simulink model "Lgsvl_ADRC_PP"  (R2023a)
settings: Solver=VariableStepAuto  StartTime=0.0  StopTime=inf  RelTol=1e-3
values from neighbouring files (symbols this model uses):
  Caf = 140000    [ADRC_PP.m]    (also in ADRC_Pure_Pursuit.m)
  Izz = 1000    [ADRC_PP.m]    (also in ADRC_Pure_Pursuit.m)
  lf = 1.63886    [ADRC_PP.m]    (also in ADRC_Pure_Pursuit.m)
  observer_discrete = c2d(observer, T)    [ADRC_PP.m]    (also in ADRC_Pure_Pursuit.m)
libraries: ros2lib x8, simulink_extras x2
settings Model: Creator=adlink  LastModifiedBy=adlink

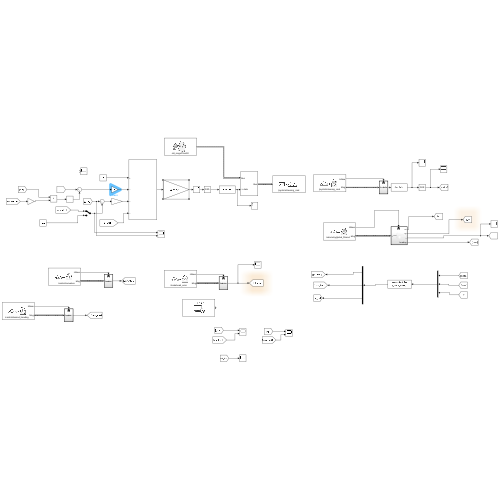
[thumbnail: Simulink's stored preview of the top-level diagram]
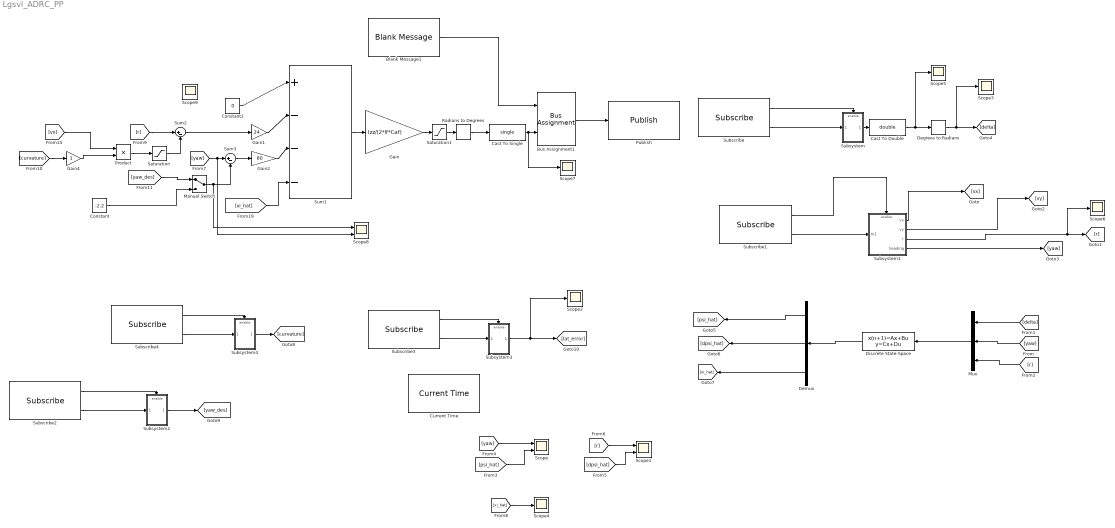
== system Lgsvl_ADRC_PP ==
  Blank Message1 : ros2lib/Blank Message  messageClass=Message  entityType=std_msgs/Float32  messageType=std_msgs/Float32  SampleTime=0.01
  Bus Assignment1 : BusAssignment  AssignedSignals=data
  Cast To Double : DataTypeConversion  OutDataTypeStr=double  SaturateOnIntegerOverflow=off  RndMeth=Floor
  Cast To Single : DataTypeConversion  OutDataTypeStr=single  SaturateOnIntegerOverflow=off  RndMeth=Floor
  Constant : Constant  Value=-2.2
  Constant2 : Constant  Value=0
  Current Time : ros2lib/Current Time  OutputFormat=bus  SampleTime=0.01  ModelName=Lgsvl_ADRC_PP
  Degrees to Radians : simulink_extras/Transformations/Degrees to Radians
  Demux : Demux  Outputs=3
  Discrete State-Space : DiscreteStateSpace  A=observer_discrete.A  B=observer_discrete.B  C=observer_discrete.C  D=observer_discrete.D  SampleTime=0.01
  Gain : Gain  Gain=Izz/(2*lf*Caf)
  Gain1 : Gain  Gain=24
  Gain2 : Gain  Gain=80
  Gain4 : Gain
  Manual Switch : ManualSwitch
  Mux : Mux  Inputs=3
  Product : Product
  Publish : ros2lib/Publish  topicSource=Select from ROS network  topic=/joystick/steering_cmd  messageType=std_msgs/Float32  QOSHistory=Keep last  QOSDepth=1  QOSReliability=Reliable  QOSDurability=Volatile
  Radians to Degrees : simulink_extras/Transformations/Radians to Degrees
  Saturation : Saturate  UpperLimit=0.2  LowerLimit=-0.2
  Saturation1 : Saturate  UpperLimit=0.3  LowerLimit=-0.3
  Scope : Scope  NumInputPorts=2
  Scope1 : Scope  NumInputPorts=2
  Scope{2..7,9} (7 alike) : Scope
  Scope8 : Scope  NumInputPorts=2
  Subscribe : ros2lib/Subscribe  topicSource=Select from ROS network  topic=/joystick/steering_cmd  messageType=std_msgs/Float32  sampleTime=0.01  QOSHistory=Keep last  QOSDepth=1  QOSReliability=Reliable  QOSDurability=Volatile
  Subscribe1 : ros2lib/Subscribe  topicSource=Select from ROS network  topic=/odometry/global_filtered  messageType=nav_msgs/Odometry  sampleTime=0.01  QOSHistory=Keep last  QOSDepth=1  QOSReliability=Reliable  QOSDurability=Volatile
  Subscribe2 : ros2lib/Subscribe  topicSource=Select from ROS network  topic=/control/desired_heading  messageType=std_msgs/Float32  sampleTime=0.01  QOSHistory=Keep last  QOSDepth=1  QOSReliability=Reliable  QOSDurability=Volatile
  Subscribe3 : ros2lib/Subscribe  topicSource=Select from ROS network  topic=/lookahead_error  messageType=std_msgs/Float64  sampleTime=0.01  QOSHistory=Keep last  QOSDepth=1  QOSReliability=Reliable  QOSDurability=Volatile
  Subscribe4 : ros2lib/Subscribe  topicSource=Select from ROS network  topic=/control/curvature  messageType=std_msgs/Float32  sampleTime=0.01  QOSHistory=Keep last  QOSDepth=1  QOSReliability=Reliable  QOSDurability=Volatile
  Subsystem : Subsystem
  Subsystem1 : Subsystem
  Subsystem2 : Subsystem
  Subsystem3 : Subsystem
  Subsystem4 : Subsystem
  Sum1 : Sum  Inputs=|+---
  Sum2 : Sum  Inputs=|+-
  Sum3 : Sum  Inputs=|+-
  wires:
  Blank Message1/1 -> Bus Assignment1/1
  [yaw] -> Scope/1
  Gain/1 -> Saturation1/1
  Saturation1/1 -> Radians to Degrees/1
  Radians to Degrees/1 -> Cast To Single/1
  Cast To Double/1 -> Scope5/1, Degrees to Radians/1
  Subsystem1/4(heading) -> [yaw]
  Bus Assignment1/1 -> Publish/1
  [r] -> Scope1/1
  Demux/3 -> [xi_hat]
  Subscribe2/1 -> Subsystem2/Enable
  Constant2/1 -> Sum1/1
  [dpsi_hat] -> Scope1/2
  [curvature] -> Gain4/1
  [yaw] -> Scope8/2, Sum3/1
  Sum2/1 -> Gain1/1
  [xi_hat] -> Sum1/4
  Mux/1 -> Discrete State-Space/1
  Subscribe1/2 -> Subsystem1/1(In1)
  Subsystem3/1(<data>) -> Scope2/1, [lat_error]
  Degrees to Radians/1 -> Scope3/1, [delta]
  Subsystem/1(delta) -> Cast To Double/1
  [r] -> Mux/3
  [r] -> Sum2/1
  Subscribe/2 -> Subsystem/1(In1)
  Subscribe4/1 -> Subsystem4/Enable
  Subsystem1/2(vy) -> [vy]
  Demux/2 -> [dpsi_hat]
  Constant/1 -> Manual Switch/2
  [yaw] -> Mux/2
  [delta] -> Mux/1
  Subscribe1/1 -> Subsystem1/Enable
  Subscribe2/2 -> Subsystem2/1(In1)
  Subsystem4/1(<data>) -> [curvature]
  Subscribe/1 -> Subsystem/Enable
  [xi_hat] -> Scope4/1
  Subsystem2/1(<data>) -> [yaw_des]
  Subscribe4/2 -> Subsystem4/1(In1)
  Subsystem1/3(r) -> Scope6/1, [r]
  Subscribe3/2 -> Subsystem3/1(In1)
  Cast To Single/1 -> Scope7/1, Bus Assignment1/2
  Gain4/1 -> Product/2
  Subscribe3/1 -> Subsystem3/Enable
  Discrete State-Space/1 -> Demux/1
  Subsystem1/1(vx) -> [vx]
  Sum3/1 -> Gain2/1
  Manual Switch/1 -> Scope8/1, Sum3/2
  Gain1/1 -> Sum1/2
  [psi_hat] -> Scope/2
  Gain2/1 -> Sum1/3
  Demux/1 -> [psi_hat]
  Sum1/1 -> Gain/1
  [vx] -> Product/1
  [yaw_des] -> Manual Switch/1
  Product/1 -> Saturation/1
  Saturation/1 -> Sum2/2

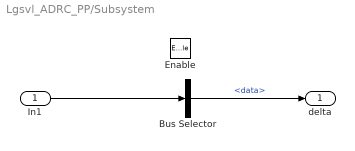
== system Lgsvl_ADRC_PP/Subsystem ==
  In1 : Inport
  Enable : EnablePort
  Bus Selector : BusSelector  OutputSignals=data
  delta : Outport
  wires:
  In1/1 -> Bus Selector/1
  Bus Selector/1 -> delta/1  "<data>"

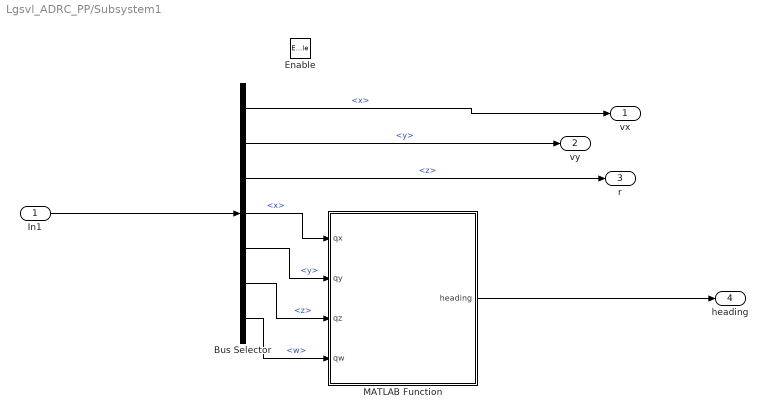
== system Lgsvl_ADRC_PP/Subsystem1 ==
  In1 : Inport
  Enable : EnablePort
  Bus Selector : BusSelector  OutputSignals=twist.twist.linear.x,twist.twist.linear.y,twist.twist.angular.z,pose.pose.orientation.x,pose.pose.orientation.y,pose.pose.orientation.z,pose.pose.orientation.w
  MATLAB Function : MATLAB Function  TreatAsAtomicUnit=on
  vx : Outport
  vy : Outport  Port=2
  r : Outport  Port=3
  heading : Outport  Port=4
  wires:
  Bus Selector/4 -> MATLAB Function/1(qx)  "<x>"
  Bus Selector/3 -> r/1  "<z>"
  Bus Selector/7 -> MATLAB Function/4(qw)  "<w>"
  MATLAB Function/1(heading) -> heading/1
  Bus Selector/5 -> MATLAB Function/2(qy)  "<y>"
  Bus Selector/2 -> vy/1  "<y>"
  In1/1 -> Bus Selector/1
  Bus Selector/6 -> MATLAB Function/3(qz)  "<z>"
  Bus Selector/1 -> vx/1  "<x>"

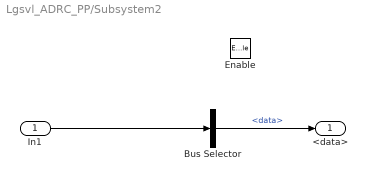
== system Lgsvl_ADRC_PP/Subsystem2 ==
  In1 : Inport
  Enable : EnablePort
  Bus Selector : BusSelector  OutputSignals=data
  <data> : Outport
  wires:
  In1/1 -> Bus Selector/1
  Bus Selector/1 -> <data>/1  "<data>"

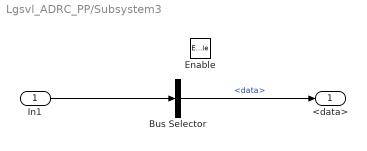
== system Lgsvl_ADRC_PP/Subsystem3 ==
  In1 : Inport
  Enable : EnablePort
  Bus Selector : BusSelector  OutputSignals=data
  <data> : Outport
  wires:
  In1/1 -> Bus Selector/1
  Bus Selector/1 -> <data>/1  "<data>"

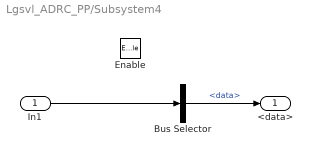
== system Lgsvl_ADRC_PP/Subsystem4 ==
  In1 : Inport
  Enable : EnablePort
  Bus Selector : BusSelector  OutputSignals=data
  <data> : Outport
  wires:
  In1/1 -> Bus Selector/1
  Bus Selector/1 -> <data>/1  "<data>"

== matlab function Lgsvl_ADRC_PP/Subsystem1/MATLAB Function ==
  data: qx input; heading output; qy input; qz input; qw input
function heading = fcn(qx, qy, qz, qw)
siny_cosp = 2.0 * (qw * qz + qx * qy);
cosy_cosp = 1.0 - 2.0 * (qy * qy + qz * qz);
heading = atan2(siny_cosp, cosy_cosp);
